simulink model "Arm_cobot"  (Simulink 8.3)
settings: Solver=ode1  StartTime=0.0  StopTime=inf  FixedStep=TA  RelTol=1e-3
PreLoadFcn:
  | startup
  | gui_starter
  | init_starter
PostLoadFcn:
  | init_check
InitFcn:
  | init_starter
undefined symbols (not defined in the file): alphaM, alphaT, Arm7ConLib, Arms2, baseOffset_x, baseOffset_y, baseOffset_z, betaM, betaT, cobotNa, cobotNb, D1, D2, D3, D4, D5, D6, D7, d_FTS_EE_L, d_FTS_EE_R, DD1, DD2, DD3, DD4, DD5, DD6, DD7, Do, Dp, EEL, EER, Fcal_L, Fcal_R, I1, I2, I3, I4, I5, I6, I7, IFL, IFR, impuls2rad_L, impuls2rad_R, Inert_L, Inert_R, KdC, KiC, Ko, Kp, KpC, LTool_L, LTool_R, mEE_L, mEE_R, Mo, Mp, P1, P2, P3 ... (+28)
libraries: sensoray x16, rtai_utilities x11, simulink x2, jr3lib x2, Interface x1
(part 3 of 3)

== system Arm_cobot/Right Arm/ForceControl/Subsystem/PII2 ==
  In_1 : Inport
  reset : Inport  Port=2
  Integrator : Integrator  ExternalReset=falling  UpperSaturationLimit=S  LowerSaturationLimit=-S
  Proportional : Gain  Gain=P  SaturateOnIntegerOverflow=on  OutDataTypeStr=Inherit: Same as input  ParamDataTypeStr=Inherit: Same as input
  Saturation : Saturate  UpperLimit=S  LowerLimit=-S
  Sum : Sum  SaturateOnIntegerOverflow=on  InputSameDT=on  OutDataTypeStr=Inherit: Same as first input
  Sum1 : Sum  Inputs=-+|
  Sum2 : Sum  Inputs=|++
  Out_1 : Outport  InitialOutput=0
  wires:
  Proportional/1 -> Sum/1
  Integrator/1 -> Sum/2
  Sum/1 -> Sum1/1, Saturation/1
  Sum2/1 -> Integrator/1
  In_1/1 -> Sum2/1, Proportional/1
  Saturation/1 -> Sum1/2, Out_1/1
  Sum1/1 -> Sum2/2
  reset/1 -> Integrator/2

== system Arm_cobot/Right Arm/ForceControl/Subsystem/PII3 ==
  In_1 : Inport
  reset : Inport  Port=2
  Integrator : Integrator  ExternalReset=falling  UpperSaturationLimit=S  LowerSaturationLimit=-S
  Proportional : Gain  Gain=P  SaturateOnIntegerOverflow=on  OutDataTypeStr=Inherit: Same as input  ParamDataTypeStr=Inherit: Same as input
  Saturation : Saturate  UpperLimit=S  LowerLimit=-S
  Sum : Sum  SaturateOnIntegerOverflow=on  InputSameDT=on  OutDataTypeStr=Inherit: Same as first input
  Sum1 : Sum  Inputs=-+|
  Sum2 : Sum  Inputs=|++
  Out_1 : Outport  InitialOutput=0
  wires:
  Proportional/1 -> Sum/1
  Integrator/1 -> Sum/2
  Sum/1 -> Sum1/1, Saturation/1
  Sum2/1 -> Integrator/1
  In_1/1 -> Sum2/1, Proportional/1
  Saturation/1 -> Sum1/2, Out_1/1
  Sum1/1 -> Sum2/2
  reset/1 -> Integrator/2

== system Arm_cobot/Right Arm/ForceControl/Subsystem/PII4 ==
  In_1 : Inport
  reset : Inport  Port=2
  Integrator : Integrator  ExternalReset=falling  UpperSaturationLimit=S  LowerSaturationLimit=-S
  Proportional : Gain  Gain=P  SaturateOnIntegerOverflow=on  OutDataTypeStr=Inherit: Same as input  ParamDataTypeStr=Inherit: Same as input
  Saturation : Saturate  UpperLimit=S  LowerLimit=-S
  Sum : Sum  SaturateOnIntegerOverflow=on  InputSameDT=on  OutDataTypeStr=Inherit: Same as first input
  Sum1 : Sum  Inputs=-+|
  Sum2 : Sum  Inputs=|++
  Out_1 : Outport  InitialOutput=0
  wires:
  Proportional/1 -> Sum/1
  Integrator/1 -> Sum/2
  Sum/1 -> Sum1/1, Saturation/1
  Sum2/1 -> Integrator/1
  In_1/1 -> Sum2/1, Proportional/1
  Saturation/1 -> Sum1/2, Out_1/1
  Sum1/1 -> Sum2/2
  reset/1 -> Integrator/2

== system Arm_cobot/Right Arm/ForceControl/Subsystem/PII5 ==
  In_1 : Inport
  reset : Inport  Port=2
  Integrator : Integrator  ExternalReset=falling  UpperSaturationLimit=S  LowerSaturationLimit=-S
  Proportional : Gain  Gain=P  SaturateOnIntegerOverflow=on  OutDataTypeStr=Inherit: Same as input  ParamDataTypeStr=Inherit: Same as input
  Saturation : Saturate  UpperLimit=S  LowerLimit=-S
  Sum : Sum  SaturateOnIntegerOverflow=on  InputSameDT=on  OutDataTypeStr=Inherit: Same as first input
  Sum1 : Sum  Inputs=-+|
  Sum2 : Sum  Inputs=|++
  Out_1 : Outport  InitialOutput=0
  wires:
  Proportional/1 -> Sum/1
  Integrator/1 -> Sum/2
  Sum/1 -> Sum1/1, Saturation/1
  Sum2/1 -> Integrator/1
  In_1/1 -> Sum2/1, Proportional/1
  Saturation/1 -> Sum1/2, Out_1/1
  Sum1/1 -> Sum2/2
  reset/1 -> Integrator/2

== system Arm_cobot/Right Arm/Impedance equation RIGHT/Impedance  Equation/Subsystem ==
  In1 : Inport
  Demux : Demux  Outputs=[1,3]
  Demux1 : Demux  Outputs=[3,3,3]
  Dot Product : DotProduct  InputSameDT=on  OutDataTypeStr=Inherit: Inherit via internal rule
  Dot Product1 : DotProduct  InputSameDT=on  OutDataTypeStr=Inherit: Inherit via internal rule
  Dot Product2 : DotProduct  InputSameDT=on  OutDataTypeStr=Inherit: Inherit via internal rule
  Gain2 : Gain  Gain=K_o  Multiplication=Matrix(K*u)  OutDataTypeStr=Inherit: Same as input  ParamDataTypeStr=Inherit: Same as input
  Mux2 : Mux  Inputs=3
  Subsystem3 : Subsystem
      mask Display: disp('2tr(E)')
  Terminator : Terminator
  Out1 : Outport
  wires:
  In1/1 -> Subsystem3/1(In1), Demux/1
  Subsystem3/1(Out1) -> Demux1/1
  Demux/2 -> Gain2/1
  Demux/1 -> Terminator/1
  Dot Product/1 -> Mux2/3
  Dot Product1/1 -> Mux2/2
  Dot Product2/1 -> Mux2/1
  Demux1/1 -> Dot Product2/1
  Demux1/2 -> Dot Product1/1
  Demux1/3 -> Dot Product/1
  Mux2/1 -> Out1/1
  Gain2/1 -> Dot Product/2, Dot Product1/2, Dot Product2/2

== system Arm_cobot/Right Arm/Impedance equation RIGHT/Impedance  Equation/Subsystem1 ==
  note: angular vel.
  note: dQ_dc
  Q_dc : Inport
  w_dc : Inport  Port=2
  Mux : Mux  Inputs=[3, 4]
  S-Function : S-Function  FunctionName=Qprop_S  EnableBusSupport=off
  Out1 : Outport
  wires:
  Q_dc/1 -> Mux/2
  Mux/1 -> S-Function/1
  w_dc/1 -> Mux/1
  S-Function/1 -> Out1/1

== system Arm_cobot/Right Arm/Impedance equation RIGHT/Impedance  Equation/Subsystem2 ==
  Q_2 : Inport
  Q_1 : Inport  Port=2
  Mux : Mux  Inputs=2
  S-Function : S-Function  FunctionName=Qproduct_S  EnableBusSupport=off
  Out1 : Outport
  wires:
  Q_1/1 -> Mux/1
  Q_2/1 -> Mux/2
  Mux/1 -> S-Function/1
  S-Function/1 -> Out1/1

== system Arm_cobot/Right Arm/Impedance equation RIGHT/Impedance  Equation/Subsystem3 ==
  In1 : Inport
  Constant : Constant  Value=zeros(1,3)
  Switch : Switch  Threshold=.5
  Out1 : Outport
  wires:
  In1/1 -> Switch/1
  [RCpl] -> Switch/2
  Switch/1 -> Out1/1
  Constant/1 -> Switch/3

== system Arm_cobot/Right Arm/Impedance equation RIGHT/Impedance  Equation/Subsystem4 ==
  In1 : Inport
  Constant : Constant  Value=zeros(1,3)
  Switch : Switch  Threshold=.5
  Out1 : Outport
  wires:
  In1/1 -> Switch/1
  [RCpl] -> Switch/2
  Switch/1 -> Out1/1
  Constant/1 -> Switch/3

== system Arm_cobot/Right Arm/Impedance equation RIGHT/Impedance  Equation/Subsystem6 ==
  In1 : Inport
  Constant : Constant  Value=zeros(1,4)
  Switch : Switch  Threshold=.5
  Out1 : Outport
  wires:
  In1/1 -> Switch/1
  [RCpl] -> Switch/2
  Switch/1 -> Out1/1
  Constant/1 -> Switch/3

== system Arm_cobot/Right Arm/Impedance equation RIGHT/Impedance  Equation/Subsystem7 ==
  In1 : Inport
  Constant : Constant  Value=zeros(1,3)
  Switch : Switch  Threshold=.5
  Out1 : Outport
  wires:
  In1/1 -> Switch/1
  [RCpl] -> Switch/2
  Switch/1 -> Out1/1
  Constant/1 -> Switch/3

== system Arm_cobot/Right Arm/Inverse kinematics RIGHT/IK_R weighted damped least square/PID ==
  In : Inport
  D value : Gain  Gain=KdC
  Derivative : Derivative
  I value : Gain  Gain=KiC
  Integrator : Integrator
  P value : Gain  Gain=KpC
  Saturation : Saturate  UpperLimit=10  LowerLimit=-10
  Sum2 : Sum  Inputs=+++
  Out : Outport
  wires:
  Sum2/1 -> Out/1
  Derivative/1 -> D value/1
  Integrator/1 -> I value/1
  In/1 -> Derivative/1, Integrator/1, P value/1
  I value/1 -> Saturation/1
  P value/1 -> Sum2/1
  Saturation/1 -> Sum2/2
  D value/1 -> Sum2/3

== system Arm_cobot/Right Arm/Inverse kinematics RIGHT/IK_R weighted damped least square/Quaternion to  angular velocity ==
  Q : Inport
  Derivative1 : Derivative
  Mux : Mux  Inputs=2
  S-Function1 : S-Function  FunctionName=Q2AngVel_S  EnableBusSupport=off
  W : Outport
  wires:
  Derivative1/1 -> Mux/2
  Mux/1 -> S-Function1/1
  Q/1 -> Derivative1/1, Mux/1
  S-Function1/1 -> W/1

== system Arm_cobot/Right Arm/Inverse kinematics RIGHT/IK_R weighted damped least square/WDLS ==
  XR_dot : Inport
  qR : Inport  Port=2
  Anti Windup : MATLAB Function  TreatAsAtomicUnit=on
  Jacobian : S-Function  FunctionName=j_S  EnableBusSupport=off
  LTCP : Constant  Value=LTool_R
  Math Function : Math  Operator=transpose  SaturateOnIntegerOverflow=on
  Mux : Mux  Inputs=2
  Reshape : Reshape  OutputDimensionality=Customize  OutputDimensions=[7,7]
  WDLS right : MATLAB Function  TreatAsAtomicUnit=on
  q'2q : Integrator  InitialCondition=qIR
  q_damp : Outport
  wires:
  Mux/1 -> Jacobian/1
  LTCP/1 -> Mux/1
  qR/1 -> Mux/2, WDLS right/3(q), Anti Windup/2(q)
  Jacobian/1 -> Reshape/1
  Reshape/1 -> Math Function/1
  q'2q/1 -> q_damp/1
  Math Function/1 -> WDLS right/1(jacobian)
  XR_dot/1 -> WDLS right/2(xDot)
  WDLS right/1(qDot) -> Anti Windup/1(qDot)
  Anti Windup/1(qDot1) -> q'2q/1

== system Arm_cobot/Right Arm/PD Joint Control  RIGHT/PID Digital Derivative1/PID + digital Derivative1 ==
  In_1 : Inport
  Discrete Transfer Fcn : DiscreteTransferFcn  Numerator=[1 -1]  Denominator=TA*[1 0]  SampleTime=TA
  Integral : TransferFcn  Numerator=[I]  Denominator=[1 0]
  Proportional : Gain  Gain=P  SaturateOnIntegerOverflow=on  OutDataTypeStr=Inherit: Same as input  ParamDataTypeStr=Inherit: Same as input
  Proportional1 : Gain  Gain=D  SaturateOnIntegerOverflow=on  OutDataTypeStr=Inherit: Same as input  ParamDataTypeStr=Inherit: Same as input
  Sum : Sum  Inputs=+++  SaturateOnIntegerOverflow=on  InputSameDT=on  OutDataTypeStr=Inherit: Same as first input
  Out_1 : Outport  InitialOutput=0
  wires:
  Proportional1/1 -> Discrete Transfer Fcn/1
  Proportional/1 -> Sum/1
  Integral/1 -> Sum/2
  Discrete Transfer Fcn/1 -> Sum/3
  In_1/1 -> Proportional/1, Integral/1, Proportional1/1
  Sum/1 -> Out_1/1

== system Arm_cobot/Right Arm/PD Joint Control  RIGHT/PID Digital Derivative1/PID + digital Derivative2 ==
  In_1 : Inport
  Discrete Transfer Fcn : DiscreteTransferFcn  Numerator=[1 -1]  Denominator=TA*[1 0]  SampleTime=TA
  Integral : TransferFcn  Numerator=[I]  Denominator=[1 0]
  Proportional : Gain  Gain=P  SaturateOnIntegerOverflow=on  OutDataTypeStr=Inherit: Same as input  ParamDataTypeStr=Inherit: Same as input
  Proportional1 : Gain  Gain=D  SaturateOnIntegerOverflow=on  OutDataTypeStr=Inherit: Same as input  ParamDataTypeStr=Inherit: Same as input
  Sum : Sum  Inputs=+++  SaturateOnIntegerOverflow=on  InputSameDT=on  OutDataTypeStr=Inherit: Same as first input
  Out_1 : Outport  InitialOutput=0
  wires:
  Sum/1 -> Out_1/1
  In_1/1 -> Proportional1/1, Integral/1, Proportional/1
  Discrete Transfer Fcn/1 -> Sum/3
  Integral/1 -> Sum/2
  Proportional/1 -> Sum/1
  Proportional1/1 -> Discrete Transfer Fcn/1

== system Arm_cobot/Right Arm/PD Joint Control  RIGHT/PID Digital Derivative1/PID + digital Derivative3 ==
  In_1 : Inport
  Discrete Transfer Fcn : DiscreteTransferFcn  Numerator=[1 -1]  Denominator=TA*[1 0]  SampleTime=TA
  Integral : TransferFcn  Numerator=[I]  Denominator=[1 0]
  Proportional : Gain  Gain=P  SaturateOnIntegerOverflow=on  OutDataTypeStr=Inherit: Same as input  ParamDataTypeStr=Inherit: Same as input
  Proportional1 : Gain  Gain=D  SaturateOnIntegerOverflow=on  OutDataTypeStr=Inherit: Same as input  ParamDataTypeStr=Inherit: Same as input
  Sum : Sum  Inputs=+++  SaturateOnIntegerOverflow=on  InputSameDT=on  OutDataTypeStr=Inherit: Same as first input
  Out_1 : Outport  InitialOutput=0
  wires:
  Sum/1 -> Out_1/1
  In_1/1 -> Proportional1/1, Integral/1, Proportional/1
  Discrete Transfer Fcn/1 -> Sum/3
  Integral/1 -> Sum/2
  Proportional/1 -> Sum/1
  Proportional1/1 -> Discrete Transfer Fcn/1

== system Arm_cobot/Right Arm/PD Joint Control  RIGHT/PID Digital Derivative1/PID + digital Derivative4 ==
  In_1 : Inport
  Discrete Transfer Fcn : DiscreteTransferFcn  Numerator=[1 -1]  Denominator=TA*[1 0]  SampleTime=TA
  Integral : TransferFcn  Numerator=[I]  Denominator=[1 0]
  Proportional : Gain  Gain=P  SaturateOnIntegerOverflow=on  OutDataTypeStr=Inherit: Same as input  ParamDataTypeStr=Inherit: Same as input
  Proportional1 : Gain  Gain=D  SaturateOnIntegerOverflow=on  OutDataTypeStr=Inherit: Same as input  ParamDataTypeStr=Inherit: Same as input
  Sum : Sum  Inputs=+++  SaturateOnIntegerOverflow=on  InputSameDT=on  OutDataTypeStr=Inherit: Same as first input
  Out_1 : Outport  InitialOutput=0
  wires:
  Proportional1/1 -> Discrete Transfer Fcn/1
  Proportional/1 -> Sum/1
  Integral/1 -> Sum/2
  Discrete Transfer Fcn/1 -> Sum/3
  In_1/1 -> Proportional/1, Integral/1, Proportional1/1
  Sum/1 -> Out_1/1

== system Arm_cobot/Right Arm/PD Joint Control  RIGHT/PID Digital Derivative1/PID + digital Derivative5 ==
  In_1 : Inport
  Discrete Transfer Fcn : DiscreteTransferFcn  Numerator=[1 -1]  Denominator=TA*[1 0]  SampleTime=TA
  Integral : TransferFcn  Numerator=[I]  Denominator=[1 0]
  Proportional : Gain  Gain=P  SaturateOnIntegerOverflow=on  OutDataTypeStr=Inherit: Same as input  ParamDataTypeStr=Inherit: Same as input
  Proportional1 : Gain  Gain=D  SaturateOnIntegerOverflow=on  OutDataTypeStr=Inherit: Same as input  ParamDataTypeStr=Inherit: Same as input
  Sum : Sum  Inputs=+++  SaturateOnIntegerOverflow=on  InputSameDT=on  OutDataTypeStr=Inherit: Same as first input
  Out_1 : Outport  InitialOutput=0
  wires:
  Sum/1 -> Out_1/1
  In_1/1 -> Proportional1/1, Integral/1, Proportional/1
  Discrete Transfer Fcn/1 -> Sum/3
  Integral/1 -> Sum/2
  Proportional/1 -> Sum/1
  Proportional1/1 -> Discrete Transfer Fcn/1

== system Arm_cobot/Right Arm/PD Joint Control  RIGHT/PID Digital Derivative1/PID + digital Derivative6 ==
  In_1 : Inport
  Discrete Transfer Fcn : DiscreteTransferFcn  Numerator=[1 -1]  Denominator=TA*[1 0]  SampleTime=TA
  Integral : TransferFcn  Numerator=[I]  Denominator=[1 0]
  Proportional : Gain  Gain=P  SaturateOnIntegerOverflow=on  OutDataTypeStr=Inherit: Same as input  ParamDataTypeStr=Inherit: Same as input
  Proportional1 : Gain  Gain=D  SaturateOnIntegerOverflow=on  OutDataTypeStr=Inherit: Same as input  ParamDataTypeStr=Inherit: Same as input
  Sum : Sum  Inputs=+++  SaturateOnIntegerOverflow=on  InputSameDT=on  OutDataTypeStr=Inherit: Same as first input
  Out_1 : Outport  InitialOutput=0
  wires:
  Proportional1/1 -> Discrete Transfer Fcn/1
  Proportional/1 -> Sum/1
  Integral/1 -> Sum/2
  Discrete Transfer Fcn/1 -> Sum/3
  In_1/1 -> Proportional/1, Integral/1, Proportional1/1
  Sum/1 -> Out_1/1

== system Arm_cobot/Right Arm/PD Joint Control  RIGHT/PID Digital Derivative1/PID + digital Derivative7 ==
  In_1 : Inport
  Discrete Transfer Fcn : DiscreteTransferFcn  Numerator=[1 -1]  Denominator=TA*[1 0]  SampleTime=TA
  Integral : TransferFcn  Numerator=[I]  Denominator=[1 0]
  Proportional : Gain  Gain=P  SaturateOnIntegerOverflow=on  OutDataTypeStr=Inherit: Same as input  ParamDataTypeStr=Inherit: Same as input
  Proportional1 : Gain  Gain=D  SaturateOnIntegerOverflow=on  OutDataTypeStr=Inherit: Same as input  ParamDataTypeStr=Inherit: Same as input
  Sum : Sum  Inputs=+++  SaturateOnIntegerOverflow=on  InputSameDT=on  OutDataTypeStr=Inherit: Same as first input
  Out_1 : Outport  InitialOutput=0
  wires:
  Sum/1 -> Out_1/1
  In_1/1 -> Proportional1/1, Integral/1, Proportional/1
  Discrete Transfer Fcn/1 -> Sum/3
  Integral/1 -> Sum/2
  Proportional/1 -> Sum/1
  Proportional1/1 -> Discrete Transfer Fcn/1

== system Arm_cobot/Right Arm/Right Arm/Arms/Analog Output1 ==
  In2 : Inport
  Analog Output : sensoray/Analog Output  BoardNumber=0  Channels=[0 1 2 3]  InitialOutputs=[0 0 0 0]  FinalOutputs=[0 0 0 0]  SampleTime=-1
  Analog Output1 : sensoray/Analog Output  BoardNumber=1  Channels=[0 1 2]  InitialOutputs=[0 0 0]  FinalOutputs=[0 0 0]  SampleTime=-1
  Demux : Demux  Outputs=2
  wires:
  In2/1 -> Demux/1
  Demux/1 -> Analog Output/1
  Demux/2 -> Analog Output1/1

== system Arm_cobot/Right Arm/Right Arm/Arms/Encoder Input1 ==
  Encoder Input : sensoray/Encoder Input  BoardNumber=0  Channels=[0 2 3 5]  InitialValues=[0 0 0 0]  SampleTime=simget(bdroot,'FixedStep')  ResetEncoder=off
  Encoder Input1 : sensoray/Encoder Input  BoardNumber=1  Channels=[0 2 3]  InitialValues=[0 0 0]  SampleTime=simget(bdroot,'FixedStep')  ResetEncoder=off
  Mux : Mux  Inputs=2
  Out1 : Outport
  wires:
  Encoder Input/1 -> Mux/1
  Encoder Input1/1 -> Mux/2
  Mux/1 -> Out1/1

== system Arm_cobot/Right Arm/Right Arm/Arms/Pose A offset1 ==
  in : Inport
  Constant : Constant  Value=pi/2
  Constant1 : Constant  Value=0
  Constant2 : Constant  Value=0
  Demux : Demux  Outputs=7
  Mux : Mux  Inputs=7
  Sum : Sum  Inputs=++|  SaturateOnIntegerOverflow=on  InputSameDT=on  OutDataTypeStr=Inherit: Same as first input
  Sum1 : Sum  Inputs=++|  SaturateOnIntegerOverflow=on  InputSameDT=on  OutDataTypeStr=Inherit: Same as first input
  Sum2 : Sum  Inputs=++|  SaturateOnIntegerOverflow=on  InputSameDT=on  OutDataTypeStr=Inherit: Same as first input
  out : Outport
  wires:
  Mux/1 -> out/1
  in/1 -> Demux/1
  Demux/4 -> Mux/4
  Sum1/1 -> Mux/3
  Constant1/1 -> Sum1/1
  Demux/3 -> Sum1/2
  Sum/1 -> Mux/2
  Demux/2 -> Sum/2
  Constant/1 -> Sum/1
  Demux/1 -> Mux/1
  Demux/5 -> Mux/5
  Demux/6 -> Mux/6
  Sum2/1 -> Mux/7
  Constant2/1 -> Sum2/1
  Demux/7 -> Sum2/2

== system Arm_cobot/Right Arm/Right Arm/Arms/fts2cart right ==
  q : Inport
  Fmes/Tmes : Inport  Port=2
  Constant : Constant  Value=Fcal
  Constant1 : Constant  Value=LTCP
  Constant2 : Constant  Value=LEE
  Constant3 : Constant  Value=MEE
  Constant4 : Constant  Value=OFFbee
  Constant5 : Constant  Value=Tcal
  Demux : Demux  Outputs=2
  Mux : Mux  Inputs=9
  S-Function : S-Function  FunctionName=fts2cart_r_S  EnableBusSupport=off
  Torques have to be divided  through 10 : Gain  Gain=1/10
  F/T : Outport
  wires:
  Torques have to be divided  through 10/1 -> Mux/9
  Mux/1 -> S-Function/1
  S-Function/1 -> F/T/1
  Fmes/Tmes/1 -> Demux/1
  q/1 -> Mux/7
  Constant5/1 -> Mux/8
  Demux/2 -> Torques have to be divided  through 10/1
  Constant2/1 -> Mux/1
  Constant1/1 -> Mux/2
  Constant3/1 -> Mux/3
  Constant4/1 -> Mux/4
  Constant/1 -> Mux/5
  Demux/1 -> Mux/6

== system Arm_cobot/Left Arm/Impedance equation LEFT/Impedance  Equation/Subsystem/Subsystem3 ==
  In1 : Inport
  Constant : Constant  Value=0
  Constant1 : Constant  Value=0
  Demux1 : Demux  Outputs=[1,3]
  Demux2 : Demux  Outputs=3
  Gain : Gain  Gain=-1  SaturateOnIntegerOverflow=on  OutDataTypeStr=Inherit: Same as input  ParamDataTypeStr=Inherit: Same as input
  Gain1 : Gain  Gain=-1  SaturateOnIntegerOverflow=on  OutDataTypeStr=Inherit: Same as input  ParamDataTypeStr=Inherit: Same as input
  Gain2 : Gain  Gain=-1  SaturateOnIntegerOverflow=on  OutDataTypeStr=Inherit: Same as input  ParamDataTypeStr=Inherit: Same as input
  Gain3 : Gain  Gain=2  SaturateOnIntegerOverflow=on  OutDataTypeStr=Inherit: Same as input  ParamDataTypeStr=Inherit: Same as input
  Mux1 : Mux  Inputs=9
  Mux2 : Mux  Inputs=9
  Sum : Sum  Inputs=|+-  SaturateOnIntegerOverflow=on  InputSameDT=on  OutDataTypeStr=Inherit: Same as first input
  Out1 : Outport
  wires:
  In1/1 -> Demux1/1
  Sum/1 -> Gain3/1
  Gain2/1 -> Mux2/8
  Demux2/1 -> Gain2/1, Mux2/6
  Gain1/1 -> Mux2/4
  Demux2/2 -> Mux2/7, Gain/1
  Gain/1 -> Mux2/3
  Demux2/3 -> Gain1/1, Mux2/2
  Constant1/1 -> Mux2/9, Mux2/5, Mux2/1
  Mux2/1 -> Sum/2
  Mux1/1 -> Sum/1
  Demux1/1 -> Mux1/9, Mux1/1, Mux1/5
  Constant/1 -> Mux1/8, Mux1/7, Mux1/6, Mux1/4, Mux1/3, Mux1/2
  Demux1/2 -> Demux2/1
  Gain3/1 -> Out1/1

== system Arm_cobot/Right Arm/Impedance equation RIGHT/Impedance  Equation/Subsystem/Subsystem3 ==
  In1 : Inport
  Constant : Constant  Value=0
  Constant1 : Constant  Value=0
  Demux1 : Demux  Outputs=[1,3]
  Demux2 : Demux  Outputs=3
  Gain : Gain  Gain=-1  SaturateOnIntegerOverflow=on  OutDataTypeStr=Inherit: Same as input  ParamDataTypeStr=Inherit: Same as input
  Gain1 : Gain  Gain=-1  SaturateOnIntegerOverflow=on  OutDataTypeStr=Inherit: Same as input  ParamDataTypeStr=Inherit: Same as input
  Gain2 : Gain  Gain=-1  SaturateOnIntegerOverflow=on  OutDataTypeStr=Inherit: Same as input  ParamDataTypeStr=Inherit: Same as input
  Gain3 : Gain  Gain=2  SaturateOnIntegerOverflow=on  OutDataTypeStr=Inherit: Same as input  ParamDataTypeStr=Inherit: Same as input
  Mux1 : Mux  Inputs=9
  Mux2 : Mux  Inputs=9
  Sum : Sum  Inputs=|+-  SaturateOnIntegerOverflow=on  InputSameDT=on  OutDataTypeStr=Inherit: Same as first input
  Out1 : Outport
  wires:
  In1/1 -> Demux1/1
  Sum/1 -> Gain3/1
  Gain2/1 -> Mux2/8
  Demux2/1 -> Gain2/1, Mux2/6
  Gain1/1 -> Mux2/4
  Demux2/2 -> Mux2/7, Gain/1
  Gain/1 -> Mux2/3
  Demux2/3 -> Gain1/1, Mux2/2
  Constant1/1 -> Mux2/9, Mux2/5, Mux2/1
  Mux2/1 -> Sum/2
  Mux1/1 -> Sum/1
  Demux1/1 -> Mux1/9, Mux1/1, Mux1/5
  Constant/1 -> Mux1/8, Mux1/7, Mux1/6, Mux1/4, Mux1/3, Mux1/2
  Demux1/2 -> Demux2/1
  Gain3/1 -> Out1/1

== matlab function Left Arm/Inverse kinematics LEFT/pose error in task space/Embedded MATLAB Function ==
  data: errOut output double; errIn input double; qIn input double
function errOut = err(errIn, qIn)
% This block supports an embeddable subset of the MATLAB language.
% See the help menu for details. 

errOut = zeros(7,1);

% position error
errOut(1) = errIn(1);
errOut(2) = errIn(2);
errOut(3) = errIn(3);

% orientation error
if(errIn(4) < 0)
    errOut(4) = -errIn(5);
    errOut(5) = -errIn(6);
    errOut(6) = -errIn(7);
else
    errOut(4) = errIn(5);
    errOut(5) = errIn(6);
    errOut(6) = errIn(7);
end

% elbow error
if(~isfinite(errIn(8)))
    errOut(7) = 0;
else
    errOut(7) = sin(errIn(8))*abs(qIn(4));
end

== matlab function Left Arm/Inverse kinematics LEFT/IK_L weighted damped least square/WDLS/Anti Windup ==
  data: qDot input double; q input double; qDot1 output double; q_maxL parameter double; q_minL parameter double
function qDot1 = AntiWindup_L(qDot, q, q_maxL, q_minL)

qDot1 = qDot;

% anti windup 
for i = 1:7
    if q(i) >= q_maxL(i) && qDot(i) > 0
        qDot1(i) = 0;
    elseif q(i) <= q_minL(i) && qDot(i) < 0
        qDot1(i) = 0;
    end
end

== matlab function Left Arm/Feedforward/second derivative/2ndDerivative3Points ==
  data: u0 input double; y output double; u1 input double; u2 input double; TA parameter double
function y =  secondDerivative3Pt(u0,u1,u2,TA)
% This block supports an embeddable subset of the MATLAB language.
% See the help menu for details. 


 y  = (u0 - 2*u1 + u2) ./ (TA*TA);

== matlab function Right Arm/Feedforward/second derivative/2ndDerivative3Points ==
  data: u0 input double; y output double; u1 input double; u2 input double; TA parameter double
function y =  secondDerivative3Pt(u0,u1,u2,TA)
% This block supports an embeddable subset of the MATLAB language.
% See the help menu for details. 


 y  = (u0 - 2*u1 + u2) ./ (TA*TA);

== matlab function Right Arm/Inverse kinematics RIGHT/IK_R weighted damped least square/WDLS/Anti Windup ==
  data: qDot input double; q input double; qDot1 output double; q_maxR parameter double; q_minR parameter double
function qDot1 = AntiWindup_R(qDot, q, q_maxR, q_minR)

qDot1 = qDot;

% anti windup 
for i = 1:7
    if q(i) >= q_maxR(i) && qDot(i) > 0
        qDot1(i) = 0;
    elseif q(i) <= q_minR(i) && qDot(i) < 0
        qDot1(i) = 0;
    end
end

== matlab function Right Arm/Inverse kinematics RIGHT/pose error in task space/Embedded MATLAB Function ==
  data: errOut output double; errIn input double; qIn input double
function errOut = err(errIn, qIn)
% This block supports an embeddable subset of the MATLAB language.
% See the help menu for details. 

errOut = zeros(7,1);

% position error
errOut(1) = errIn(1);
errOut(2) = errIn(2);
errOut(3) = errIn(3);

% orientation error
if(errIn(4) < 0)
    errOut(4) = -errIn(5);
    errOut(5) = -errIn(6);
    errOut(6) = -errIn(7);
else
    errOut(4) = errIn(5);
    errOut(5) = errIn(6);
    errOut(6) = errIn(7);
end

% elbow error
if(~isfinite(errIn(8)))
    errOut(7) = 0;
else
    errOut(7) = sin(errIn(8))*abs(qIn(4));
end

== matlab function Left Arm/Inverse kinematics LEFT/IK_L weighted damped least square/WDLS/WDLS left ==
  data: jacobian input double; qDot output double; xDot input double; q input double; alphaT parameter double; alphaM parameter double; betaT parameter double; betaM parameter double; q_minL parameter double; q_maxL parameter double
function qDot = WDLS(jacobian, xDot, q, alphaT, alphaM, betaT, betaM, q_minL, q_maxL)
% This block supports an embeddable subset of the MATLAB language.
% See the help menu for details. 

J = jacobian;

% singular value decomposition of the jacobian
[U,S,V] = svd(J);

% calculate alpha
alpha = 0;
if(S(7,7) < alphaT)                                          % S(7,7) is the smallest singular value
    alpha = alphaM * (1 - (S(7,7)/alphaT))^2;
else
    alpha = 0;
end

% calculate beta
beta  = zeros(7,7);
for i = 1:7
    if(S(i,i) < betaT(i))
        beta(i,i) = betaM(i) * (1 - (S(i,i)/betaT(i)))^2;
    else
        beta(i,i) = 0;
    end
end

%calculate joint limit avoidance
W = zeros(7,7);
for i = 1:7
    W(i,i) = 1 + abs((q_maxL(i)-q_minL(i))^2 * (2*q(i)-q_maxL(i)-q_minL(i)) / (4 * (q_maxL(i)-q(i))^2 * (q(i)-q_minL(i))^2));
end

qDot = inv(W) * J' * inv(J*inv(W)*J' + alpha*eye(7,7) + U*beta*U') * xDot;

% if any element of the output vector is not finite, set them all to a very small value (to get out of a mathematical instability)
if(sum(~isfinite(qDot)) > 0)
    qDot = 1e-3*ones(7,1);
end

== matlab function Right Arm/Inverse kinematics RIGHT/IK_R weighted damped least square/WDLS/WDLS right ==
  data: jacobian input double; qDot output double; xDot input double; q input double; alphaT parameter double; alphaM parameter double; betaT parameter double; betaM parameter double; q_minR parameter double; q_maxR parameter double
function qDot = WDLS(jacobian, xDot, q, alphaT, alphaM, betaT, betaM, q_minR, q_maxR)
% This block supports an embeddable subset of the MATLAB language.
% See the help menu for details. 

J = jacobian;

% singular value decomposition of the jacobian
[U,S,V] = svd(J);

% calculate alpha
alpha = 0;
if(S(7,7) < alphaT)                                          % S(7,7) is the smallest singular value
    alpha = alphaM * (1 - (S(7,7)/alphaT))^2;
else
    alpha = 0;
end

% calculate beta
beta  = zeros(7,7);
for i = 1:7
    if(S(i,i) < betaT(i))
        beta(i,i) = betaM(i) * (1 - (S(i,i)/betaT(i)))^2;
    else
        beta(i,i) = 0;
    end
end

%calculate joint limit avoidance
W = zeros(7,7);
for i = 1:7
    W(i,i) = 1 + abs((q_maxR(i)-q_minR(i))^2 * (2*q(i)-q_maxR(i)-q_minR(i)) / (4 * (q_maxR(i)-q(i))^2 * (q(i)-q_minR(i))^2));
end

qDot = inv(W) * J' * inv(J*inv(W)*J' + alpha*eye(7,7) + U*beta*U') * xDot;

% if any element of the output vector is not finite, set them all to a very small value (to get out of a mathematical instability)
if(sum(~isfinite(qDot)) > 0)
    qDot = 1e-3*ones(7,1);
end

== matlab function Interface Right/Interface Tester (sends random commands) ==
  data: y output double; xrplan input double
function y = commands(xrplan)
%#eml

persistent counter;
persistent output;

if(isempty(counter))
	counter = 0;
	output = 0;
end

counter = counter + 1;



    
y = zeros(23,1);

if(mod(counter,2000) == 0)
	output = floor(rand()*12);
end

offsetX = 0.243;
offsetY = 0;
offsetZ = 1.4;

%%initial pose
if(counter < 8000 && counter > 5100)
    output = 3;
    y(2) = offsetX + 0.5;
    y(3) = offsetY - 0.3;
    y(4) = offsetZ - 0.3;
    y(5) = 1;
    y(6) = 0;
    y(7) = 0;
    y(8) = 0;
    y(9) = 2.5;
end

if(output == 0)		output = 6;
elseif(output == 1)	output = 7;
elseif(output == 2)	output = 2;
elseif(output == 3)	output = 3;
elseif(output == 4)	output = 4;
elseif(output == 5)	output = 5;
elseif(output == 6)	output = 6;
elseif(output == 7)	output = 7;
elseif(output == 8)	output = 8;
elseif(output == 9)	output = 7;
elseif(output == 10)output = 6;
elseif(output == 11)output = 11;
elseif(output == 12)output = 11;
elseif(output == 13)output = 11;
elseif(output == 14)output = 11;
end


y(1) = output;

if(output == 2 && counter >= 4000)					% position
	y(2) = offsetX + 0.5;
	y(3) = offsetY - 0.3;
	y(4) = offsetZ - 0.35;
	y(5) = 4.9;
elseif(output == 3)				% pose
	y(2) = offsetX + 0.5;
	y(3) = offsetY - 0.3;
	y(4) = offsetZ - 0.4;
	y(5) = 1;	
	y(6) = 0;
	y(7) = 0;
	y(8) = 0;
	y(9) = 2.9;
elseif(output == 4)				% configuration
	y(2) = offsetX + 0.5;
	y(3) = offsetY - 0.3;
	y(4) = offsetZ - 0.45;
	y(5) = 1;	
	y(6) = 0;
	y(7) = 0;
	y(8) = 0;
	y(9) = 0.3;
	y(10) = 2.9;	
elseif(output == 5)				% via
	y(2) = offsetX + 0.5;
	y(3) = offsetY - 0.35;
	y(4) = offsetZ - 0.35;
	y(5) = 1;	
	y(6) = 0;
	y(7) = 0;
	y(8) = 0;
	y(9) = -0.3;
	y(10) = 2.9;	
	y(11) = 1;	
	y(12) = 1;	
elseif(output == 6)				% vel conf
	y(2) = 0.00;
	y(3) = -0.02;
	y(4) = 0.00;
	y(5) = 0.0;	
	y(6) = 0.05;
	y(7) = 0.0;
	y(8) = 0.1;		
elseif(output == 7)				% vel conf base
	y(2) = 0.00;
	y(3) = 0.02;
	y(4) = 0.00;
	y(5) = 0.0;	
	y(6) = -0.05;
	y(7) = 0.0;
	y(8) = -0.1;			
elseif(output == 8)				% via cva
	y(2) = offsetX + 0.5;
	y(3) = offsetY - 0.3;
	y(4) = offsetZ - 0.3;
	y(5) = 1;	
	y(6) = 0;
	y(7) = 0;
	y(8) = 0;
	y(9) = 0.2;
	y(10) = 0;
	y(11) = 0;
	y(12) = 0;	
	y(13) = 0;
	y(14) = 0;
	y(15) = 0;
	y(16) = 0;
	y(17) = 0;
	y(18) = 0;
	y(19) = 0;	
	y(20) = 4.9;
	y(21) = 1;
	y(22) = 1;
elseif(output == 11)			% conf feedthrough
    y(2) = xrplan(1) + 0.00001;
	y(3) = xrplan(2) + 0.00001;
	y(4) = xrplan(3) + 0.00001;
	y(5) = xrplan(4);	
	y(6) = xrplan(5);
	y(7) = xrplan(6);
	y(8) = xrplan(7);
	y(9) = xrplan(8) - 0.00001;	
end
	
end

== matlab function Interface Right/update finished flag ==
  data: out output double; in input double
function out = finished(in)

persistent logData;

numData  = 10;
out = 1;

% Initialization of logData
if(isempty(logData))
	logData = zeros(numData+1,8);										
end

logData = [in'; logData(1:numData,:)];

for i=1:numData+1
	%if(sum(logData(i,:) ~= logData(1,:)) > 0) 
	if(~(isequal(logData(i,:), logData(1,:))))
        out = 0;
		break;
	end
end


end
